simulink model "two_legged_raibert_hopper"  (R2014a)
settings: Solver=FixedStepDiscrete  StartTime=0.0  StopTime=inf  FixedStep=sample_time  RelTol=1e-3
undefined symbols (not defined in the file): A1_notch_f1, A2_notch_f1, A_lpf_accel, A_lpf_dtau, B1_lpf_accel, B1_lpf_dtau, B1_notch_f1, B2_lpf_accel, B2_lpf_dtau, B2_notch_f1, boom_height, boom_mount_angle, boom_mount_to_center_diagonal, boom_mount_to_com, contact_threshold, control_start_time, desired_torso_angle, DiscIntNeverNeededParam, dt_thrust, dx_avg_desired, dx_avg_samples, dx_desired_step, extra_leg_damping, F_thrust, fcut_contact, g, i_limit_lateral, initial_dt, j_segments, k_ff, K_notch_f1, k_placement, k_sea, kd_flight, kd_lateral, kd_leg_angle, kd_leg_length_secondary, kd_sea_torque_flight, kd_sea_torque_stance, kd_torso, kd_virtual, ki_lateral, kp_flight_max, kp_flight_min, kp_lateral, kp_leg_angle, kp_leg_length_secondary, kp_sea_torque_flight, kp_sea_torque_stance, kp_torso, kp_virtual, l0_virtual, l_boom, l_max, l_min, l_retract, l_seg, lambda1, lambda2, lateral_offset ... (+20)
libraries: simulink x14
(part 2 of 2)

== system two_legged_raibert_hopper/Control/Behavior Control/Lateral PID Control/spherical_correction_angle ==
  q_cmu : Inport
  Selector : Selector  InputPortWidth=13  Indices=[11]
  Sum1 : Sum  Inputs=|+-
  Terminator2 : Terminator
  boom_mount_angle : Constant  Value=boom_mount_angle
  lateral_correction : Gain  Gain=180/pi
  lateral_correction [rad] : Outport
  wires:
  Sum1/1 -> lateral_correction/1, lateral_correction [rad]/1
  Selector/1 -> Sum1/1  "qBoomRoll"
  q_cmu/1 -> Selector/1
  boom_mount_angle/1 -> Sum1/2
  lateral_correction/1 -> Terminator2/1

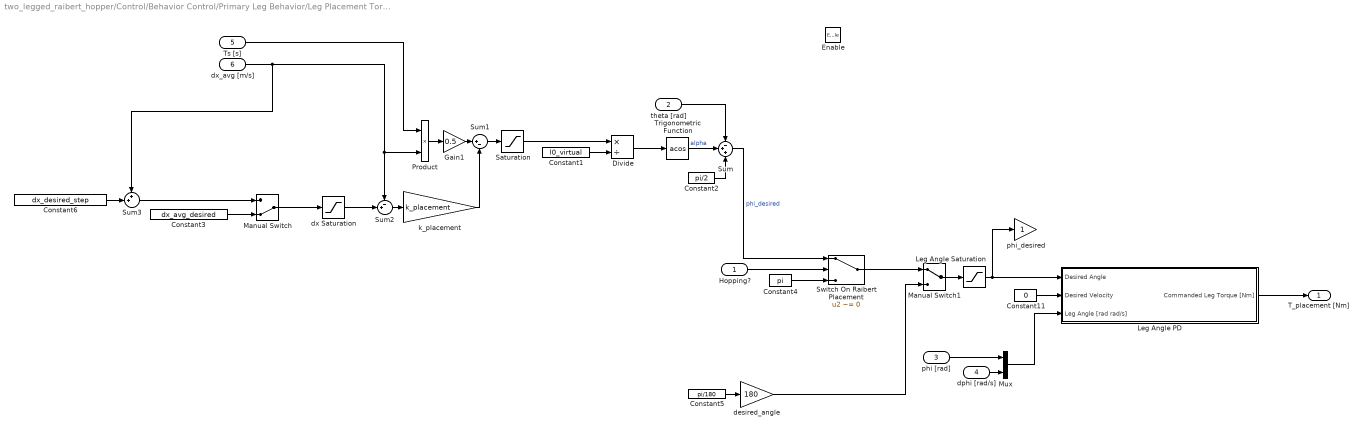
== system two_legged_raibert_hopper/Control/Behavior Control/Primary Leg Behavior/Leg Placement Torque ==
  Hopping? : Inport
  theta [rad] : Inport  Port=2
  phi [rad] : Inport  Port=3
  dphi [rad/s] : Inport  Port=4
  Ts [s] : Inport  Port=5
  dx_avg [m/s] : Inport  Port=6
  Enable : EnablePort  StatesWhenEnabling=reset
  Constant1 : Constant  Value=l0_virtual
  Constant11 : Constant  Value=0
  Constant2 : Constant  Value=pi/2
  Constant3 : Constant  Value=dx_avg_desired
  Constant4 : Constant  Value=pi
  Constant5 : Constant  Value=pi/180
  Constant6 : Constant  Value=dx_desired_step
  Divide : Product  Inputs=*/
  Gain1 : Gain  Gain=0.5
  Leg Angle PD : Subsystem
  Leg Angle Saturation : Saturate  UpperLimit=max_leg_angle  LowerLimit=min_leg_angle
      settings: AttributesFormatString=Hi: %<UpperLimit>\nLo: %<LowerLimit>
  Manual Switch : ManualSwitch  CurrentSetting=0
  Manual Switch1 : ManualSwitch
  Mux : Mux  Inputs=2
  Product : Product
  Saturation : Saturate  UpperLimit=x_limit  LowerLimit=-x_limit
      settings: AttributesFormatString=Hi: %<UpperLimit>\nLo: %<LowerLimit>
  Sum : Sum  Inputs=-++
  Sum1 : Sum  Inputs=|+-
  Sum2 : Sum  Inputs=-+|
  Sum3 : Sum  Inputs=++|
  Switch On Raibert Placement : Switch  Criteria=u2 ~= 0
  Trigonometric Function : Trigonometry  Operator=acos
  desired_angle : Gain  Gain=180
  dx Saturation : Saturate  UpperLimit=dx_avg_desired  LowerLimit=0
      settings: AttributesFormatString=Hi: %<UpperLimit>\nLo: %<LowerLimit>
  k_placement : Gain  Gain=k_placement
  phi_desired : Gain
  T_placement [Nm] : Outport  OutputWhenDisabled=reset  InitialOutput=[0]
  wires:
  Constant11/1 -> Leg Angle PD/2(Desired Velocity)
  Mux/1 -> Leg Angle PD/3(Leg Angle [rad rad/s])
  Leg Angle PD/1(Commanded Leg Torque [Nm]) -> T_placement [Nm]/1
  phi [rad]/1 -> Mux/1
  dphi [rad/s]/1 -> Mux/2
  Ts [s]/1 -> Product/1
  Product/1 -> Gain1/1
  Gain1/1 -> Sum1/1
  Saturation/1 -> Divide/1
  Constant1/1 -> Divide/2
  Trigonometric Function/1 -> Sum/2  "alpha"
  Constant2/1 -> Sum/3
  theta [rad]/1 -> Sum/1
  Sum/1 -> Switch On Raibert Placement/1  "phi_desired"
  Sum1/1 -> Saturation/1
  k_placement/1 -> Sum1/2
  Sum2/1 -> k_placement/1
  dx Saturation/1 -> Sum2/2
  Constant4/1 -> Switch On Raibert Placement/3
  Hopping?/1 -> Switch On Raibert Placement/2
  Leg Angle Saturation/1 -> phi_desired/1, Leg Angle PD/1(Desired Angle)
  Constant5/1 -> desired_angle/1
  Manual Switch/1 -> dx Saturation/1
  Constant3/1 -> Manual Switch/2
  dx_avg [m/s]/1 -> Sum3/1, Sum2/1, Product/2
  Constant6/1 -> Sum3/2
  Sum3/1 -> Manual Switch/1
  Divide/1 -> Trigonometric Function/1
  Switch On Raibert Placement/1 -> Manual Switch1/1
  desired_angle/1 -> Manual Switch1/2
  Manual Switch1/1 -> Leg Angle Saturation/1

== system two_legged_raibert_hopper/Control/Behavior Control/Primary Leg Behavior/Leg Thrust ==
  Enable : EnablePort  StatesWhenEnabling=reset  ShowOutputPort=on
  F_thrust : Gain  Gain=F_thrust
  Thrust Timer : Subsystem
  thrust period? : simulink/Logic and Bit Operations/Compare To Constant  relop=<=  const=dt_thrust  OutDataTypeStr=uint8
  Thrust [N] : Outport  OutputWhenDisabled=reset  InitialOutput=[0]
  wires:
  F_thrust/1 -> Thrust [N]/1
  Thrust Timer/1(timer [s]) -> thrust period?/1
  Enable/1 -> Thrust Timer/Enable
  thrust period?/1 -> F_thrust/1

== system two_legged_raibert_hopper/Control/Behavior Control/Primary Leg Behavior/Trunk Balance PD Compensation ==
  Torso Pitch [rad rad/s] : Inport
  Enable : EnablePort  StatesWhenEnabling=reset
  Constant2 : Constant  Value=0
  Demux : Demux  Outputs=2
  Derivative Gain : Gain  Gain=kd_torso
  Gain1 : Gain  Gain=-1
  Proportional Gain : Gain  Gain=kp_torso
  Reference Lean [rad] : Constant  Value=desired_torso_angle
  Sum1 : Sum  Inputs=|+-
  Sum4 : Sum  Inputs=|+-
  Sum5 : Sum
  Commanded Torque [Nm] : Outport  OutputWhenDisabled=reset  InitialOutput=[0]
  wires:
  Gain1/1 -> Commanded Torque [Nm]/1
  Sum1/1 -> Derivative Gain/1
  Proportional Gain/1 -> Sum5/1
  Derivative Gain/1 -> Sum5/2
  Torso Pitch [rad rad/s]/1 -> Demux/1
  Sum4/1 -> Proportional Gain/1
  Demux/1 -> Sum4/2
  Reference Lean [rad]/1 -> Sum4/1
  Constant2/1 -> Sum1/1
  Demux/2 -> Sum1/2
  Sum5/1 -> Gain1/1

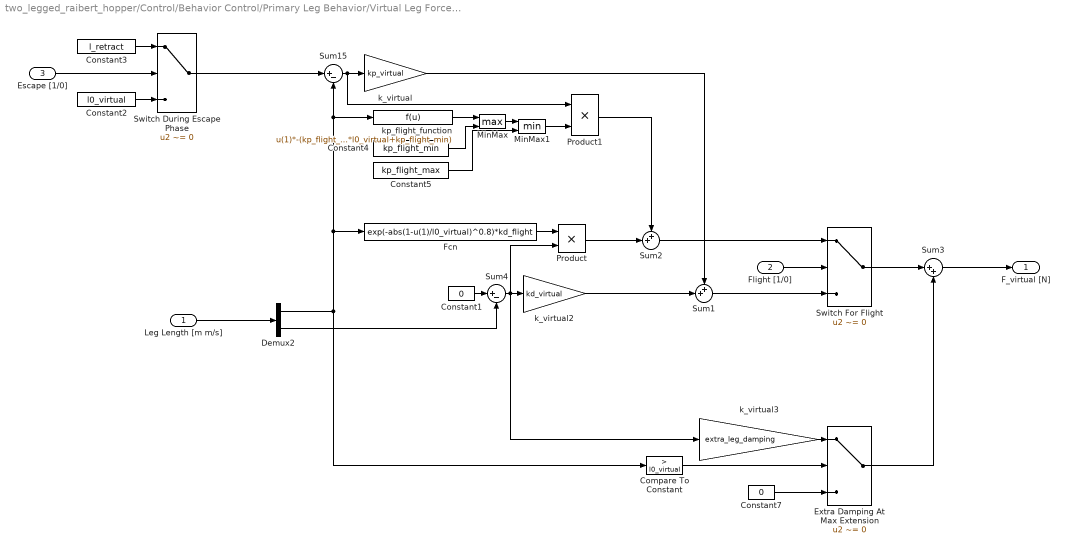
== system two_legged_raibert_hopper/Control/Behavior Control/Primary Leg Behavior/Virtual Leg Force and Swing Leg Retraction ==
  Leg Length [m m/s] : Inport
  Flight [1/0] : Inport  Port=2
  Escape [1/0] : Inport  Port=3
  Compare To Constant : simulink/Logic and Bit Operations/Compare To Constant  relop=>  const=l0_virtual  OutDataTypeStr=boolean
  Constant1 : Constant  Value=0
  Constant2 : Constant  Value=l0_virtual
  Constant3 : Constant  Value=l_retract
  Constant4 : Constant  Value=kp_flight_min
  Constant5 : Constant  Value=kp_flight_max
  Constant7 : Constant  Value=0
  Demux2 : Demux  Outputs=2
  Extra Damping At Max Extension : Switch  Criteria=u2 ~= 0
  Fcn : Fcn  Expr=exp(-abs(1-u(1)/l0_virtual)^0.8)*kd_flight
  MinMax : MinMax  Function=max  Inputs=2
  MinMax1 : MinMax  Inputs=2
  Product : Product
  Product1 : Product
  Sum1 : Sum  Inputs=++|
  Sum15 : Sum  Inputs=|+-
  Sum2 : Sum  Inputs=++|
  Sum3 : Sum  Inputs=|++
  Sum4 : Sum  Inputs=|+-
  Switch During Escape Phase : Switch  Criteria=u2 ~= 0
  Switch For Flight : Switch  Criteria=u2 ~= 0
  k_virtual : Gain  Gain=kp_virtual
  k_virtual2 : Gain  Gain=kd_virtual
  k_virtual3 : Gain  Gain=extra_leg_damping
  kp_flight_function : Fcn  Expr=u(1)*-(kp_flight_max - kp_flight_min)/(l0_virtual - l_min)+((kp_flight_max - kp_flight_min)/(l0_virtual - l_min)*l0_virtual+kp_flight_min)
  F_virtual [N] : Outport
  wires:
  Sum2/1 -> Switch For Flight/1
  Switch For Flight/1 -> Sum3/1
  Product/1 -> Sum2/2
  Constant3/1 -> Switch During Escape Phase/1
  Constant2/1 -> Switch During Escape Phase/3
  Escape [1/0]/1 -> Switch During Escape Phase/2
  Flight [1/0]/1 -> Switch For Flight/2
  k_virtual2/1 -> Sum1/2
  Sum4/1 -> k_virtual3/1, Product/2, k_virtual2/1
  k_virtual/1 -> Sum1/1
  Demux2/2 -> Sum4/2
  Constant1/1 -> Sum4/1
  Sum1/1 -> Switch For Flight/3
  Demux2/1 -> kp_flight_function/1, Sum15/2, Fcn/1, Compare To Constant/1
  Leg Length [m m/s]/1 -> Demux2/1
  Sum15/1 -> Product1/1, k_virtual/1
  Fcn/1 -> Product/1
  kp_flight_function/1 -> MinMax/1
  Product1/1 -> Sum2/1
  MinMax/1 -> MinMax1/1
  Constant4/1 -> MinMax/2
  MinMax1/1 -> Product1/2
  Constant5/1 -> MinMax1/2
  Switch During Escape Phase/1 -> Sum15/1
  Compare To Constant/1 -> Extra Damping At Max Extension/2
  Constant7/1 -> Extra Damping At Max Extension/3
  Extra Damping At Max Extension/1 -> Sum3/2
  Sum3/1 -> F_virtual [N]/1
  k_virtual3/1 -> Extra Damping At Max Extension/1

== system two_legged_raibert_hopper/Control/Behavior Control/Primary Secondary Leg Swap/Toggle ==
  Trigger : TriggerPort  TriggerType=falling  PortDimensions=1
  Logical Operator : Logic  Operator=NOT  AllPortsSameDT=off  OutDataTypeStr=boolean
  Memory : Memory  X0=1  InheritSampleTime=on
  "[1/0]" : Outport  InitialOutput=[1]
  wires:
  Memory/1 -> Logical Operator/1
  Logical Operator/1 -> Memory/1, "[1/0]"/1

== system two_legged_raibert_hopper/Control/Behavior Control/Secondary Leg Behavior/Leg Angle PD ==
  Desired Angle : Inport
  Desired Velocity : Inport  Port=2
  Leg Angle [rad rad/s] : Inport  Port=3
  Demux1 : Demux  Outputs=2
  Gain6 : Gain  Gain=kp_leg_angle
  Gain7 : Gain  Gain=kd_leg_angle
  Sum7 : Sum  Inputs=|+-
  Sum8 : Sum  Inputs=|+-
  Sum9 : Sum  Inputs=|++
  Commanded Leg Torque [Nm] : Outport
  wires:
  Leg Angle [rad rad/s]/1 -> Demux1/1
  Demux1/2 -> Sum8/2
  Gain7/1 -> Sum9/2
  Desired Angle/1 -> Sum7/1
  Sum8/1 -> Gain7/1
  Desired Velocity/1 -> Sum8/1
  Sum9/1 -> Commanded Leg Torque [Nm]/1
  Demux1/1 -> Sum7/2
  Sum7/1 -> Gain6/1
  Gain6/1 -> Sum9/1

== system two_legged_raibert_hopper/Control/Behavior Control/Secondary Leg Behavior/Leg Length PD ==
  Desired Length : Inport
  Desired Velocity : Inport  Port=2
  Leg Length [m m/s] : Inport  Port=3
  Demux1 : Demux  Outputs=2
  Sum7 : Sum  Inputs=|+-
  Sum8 : Sum  Inputs=|+-
  Sum9 : Sum
  kd_leg_length_secondary : Gain  Gain=kd_leg_length_secondary
  kp_leg_length_secondary : Gain  Gain=kp_leg_length_secondary
  Commanded Force [N] : Outport
  wires:
  kp_leg_length_secondary/1 -> Sum9/1
  Sum7/1 -> kp_leg_length_secondary/1
  Demux1/1 -> Sum7/2  "l_measured"
  Sum9/1 -> Commanded Force [N]/1
  Desired Velocity/1 -> Sum8/1
  Sum8/1 -> kd_leg_length_secondary/1
  Desired Length/1 -> Sum7/1
  kd_leg_length_secondary/1 -> Sum9/2
  Demux1/2 -> Sum8/2  "l_dot_measured"
  Leg Length [m m/s]/1 -> Demux1/1

== system two_legged_raibert_hopper/Control/Behavior Control/Velocity Estimation/Recursive Moving Average ==
  dx [m/s] : Inport
  Delay : Delay  DelayLength=dx_avg_samples  InitialCondition=0  UseCircularBuffer=on  SampleTime=sample_time
  Gain : Gain  Gain=1/dx_avg_samples
  Sum : Sum  Inputs=-++
  Unit Delay : UnitDelay  SampleTime=sample_time
  dx_avg [m/s] : Outport
  wires:
  dx [m/s]/1 -> Delay/1, Sum/2
  Sum/1 -> Gain/1, Unit Delay/1
  Delay/1 -> Sum/1
  Gain/1 -> dx_avg [m/s]/1
  Unit Delay/1 -> Sum/3

== system two_legged_raibert_hopper/Control/Behavior Control/Primary Leg Behavior/Leg Placement Torque/Leg Angle PD ==
  Desired Angle : Inport
  Desired Velocity : Inport  Port=2
  Leg Angle [rad rad/s] : Inport  Port=3
  Demux1 : Demux  Outputs=2
  Sum7 : Sum  Inputs=|+-
  Sum8 : Sum  Inputs=|+-
  Sum9 : Sum
  kd_leg_angle : Gain  Gain=kd_leg_angle
  kp_leg_angle : Gain  Gain=kp_leg_angle
  Commanded Leg Torque [Nm] : Outport
  wires:
  Leg Angle [rad rad/s]/1 -> Demux1/1
  Demux1/2 -> Sum8/2
  kd_leg_angle/1 -> Sum9/2
  Desired Angle/1 -> Sum7/1
  Sum8/1 -> kd_leg_angle/1
  Desired Velocity/1 -> Sum8/1
  Sum9/1 -> Commanded Leg Torque [Nm]/1
  Demux1/1 -> Sum7/2
  Sum7/1 -> kp_leg_angle/1
  kp_leg_angle/1 -> Sum9/1

== system two_legged_raibert_hopper/Control/Behavior Control/Primary Leg Behavior/Leg Thrust/Thrust Timer ==
  Enable : EnablePort  StatesWhenEnabling=reset  ShowOutputPort=on
  Constant : Constant
  Discrete-Time Integrator : DiscreteIntegrator  IntegratorMethod=Accumulation: Forward Euler  gainval=sample_time  ExternalReset=rising  SampleTime=sample_time  ICPrevOutput=DiscIntNeverNeededParam  ICPrevScaledInput=DiscIntNeverNeededParam
  timer [s] : Outport  InitialOutput=[0]
  wires:
  Discrete-Time Integrator/1 -> timer [s]/1
  Enable/1 -> Discrete-Time Integrator/2
  Constant/1 -> Discrete-Time Integrator/1

== stateflow chart two_legged_raibert_hopper/Control/Behavior Control/Primary Leg Behavior/Raibert  Hopper State Machine ==
  state Loading
    entry: placement = 0;
    entry: posture = 0;
    entry: thrust = 0;
    entry: flight = 0;
    entry: escape = 0;
  state Compression
    entry: placement = 0;
    entry: posture = 1;
    entry: thrust = 0;
    entry: flight = 0;
    entry: escape = 0;
  state Thrust
    entry: placement = 0;
    entry: posture = 1;
    entry: thrust = 1;
    entry: flight = 0;
    entry: escape = 0;
  state Unloading
    entry: placement = 0;
    entry: posture = 0;
    entry: thrust = 1;
    entry: flight = 0;
    entry: escape = 0;
  state Escape
    entry: placement = 0;
    entry: posture = 0;
    entry: thrust = 0;
    entry: flight = 1;
    entry: escape = 1;
  state Flight
    entry: placement = 1;
    entry: posture = 0;
    entry: thrust = 0;
    entry: flight = 1;
    entry: escape = 0;
  (junction 91) -> Loading
  Loading -> (junction 130) [order 2] : [Fy < contact_threshold]
  (junction 93) -> (junction 91)
  (junction 130) -> (junction 128)
  Loading -> Compression [order 1] : [Fy > loaded_threshold]
  (junction 115) -> Compression
  (junction 118) -> (junction 115)
  Compression -> Thrust : [dl >= 0 && dl_prev < 0]
  Thrust -> Unloading [order 1] : [Fy < loaded_threshold]
  Thrust -> (junction 102) [order 2] : [l > l_max]
  (junction 102) -> (junction 100)
  (junction 122) -> (junction 118)
  Unloading -> Escape [order 1] : [Fy < contact_threshold || l > l_max]
  Unloading -> (junction 122) [order 2] : [Fy > loaded_threshold]
  Escape -> Flight : after(t_flight,sec)
  (junction 100) -> Escape
  (default) -> Flight
  Flight -> (junction 93) : [Fy > contact_threshold]
  (junction 128) -> Flight
  data: flight output; escape output; thrust output; posture output; l input; dl input; dl_prev input; Fy input; t_flight parameter; placement output; l_max parameter; contact_threshold parameter; loaded_threshold parameter

== matlab function two_legged_raibert_hopper/Control/Behavior Control/Torque Distribution Right/Motor Torque Saturation Optimization ==
  data: x1s input; t1 output; x2s input; lambda1 parameter; lambda2 parameter; LEG_MTR_MAX_TORQUE parameter; t2 output
% Optimal leg motor torque distribution
function [t1, t2] = distribute_torque(x1s, x2s, lambda1, lambda2, LEG_MTR_MAX_TORQUE)

s = LEG_MTR_MAX_TORQUE;

% possible solutions
x1 = [                                                      x1s;
                                                            0;
                                                            s;
                                                            0;
                                                           -s;
  (lambda2*s + lambda1*x1s - lambda2*x2s)/(lambda1 + lambda2);
  (lambda1*x1s - lambda2*s + lambda2*x2s)/(lambda1 + lambda2);
  (lambda2*s + lambda1*x1s + lambda2*x2s)/(lambda1 + lambda2);
 -(lambda2*s - lambda1*x1s + lambda2*x2s)/(lambda1 + lambda2)];
 
x2 = [                                                      x2s;
                                                            s;
                                                            0;
                                                           -s;
                                                            0;
  (lambda1*s - lambda1*x1s + lambda2*x2s)/(lambda1 + lambda2);
  (lambda1*s + lambda1*x1s + lambda2*x2s)/(lambda1 + lambda2);
  (lambda1*x1s - lambda1*s + lambda2*x2s)/(lambda1 + lambda2);
 -(lambda1*s + lambda1*x1s - lambda2*x2s)/(lambda1 + lambda2)];

% test constraints
c1 = s - x1 - x2 >= 0;
c2 = s + x1 + x2 >= 0;
c3 = s - x1 + x2 >= 0;
c4 = s + x1 - x2 >= 0;
constraints = c1 & c2 & c3 & c4;

% objective function to maximize
f = -lambda1*(x1-x1s).^2-lambda2*(x2-x2s).^2;
satisfied = find(constraints);
[~,I] = max(f(satisfied));

t1 = x1(satisfied(I));
t2 = x2(satisfied(I));

== matlab function two_legged_raibert_hopper/Control/Behavior Control/Velocity Estimation/dx_from_yaw_and_roll ==
  data: qRoll input; dx output; dqYaw input; dqPitch input; l_boom parameter; boom_mount_to_center_diagonal parameter; boom_mount_to_com parameter
function dx = fcn(qRoll, dqYaw, dqPitch, l_boom, boom_mount_to_center_diagonal, boom_mount_to_com)
    dx = (l_boom+boom_mount_to_center_diagonal)*(dqYaw*cos(qRoll)) - dqPitch*boom_mount_to_com;

== matlab function two_legged_raibert_hopper/Control/Behavior Control/Torque Distribution Left/Motor Torque Saturation Optimization ==
  data: x1s input; t1 output; x2s input; lambda1 parameter; lambda2 parameter; LEG_MTR_MAX_TORQUE parameter; t2 output
% Optimal leg motor torque distribution
function [t1, t2] = distribute_torque(x1s, x2s, lambda1, lambda2, LEG_MTR_MAX_TORQUE)

s = LEG_MTR_MAX_TORQUE;

% possible solutions
x1 = [                                                      x1s;
                                                            0;
                                                            s;
                                                            0;
                                                           -s;
  (lambda2*s + lambda1*x1s - lambda2*x2s)/(lambda1 + lambda2);
  (lambda1*x1s - lambda2*s + lambda2*x2s)/(lambda1 + lambda2);
  (lambda2*s + lambda1*x1s + lambda2*x2s)/(lambda1 + lambda2);
 -(lambda2*s - lambda1*x1s + lambda2*x2s)/(lambda1 + lambda2)];
 
x2 = [                                                      x2s;
                                                            s;
                                                            0;
                                                           -s;
                                                            0;
  (lambda1*s - lambda1*x1s + lambda2*x2s)/(lambda1 + lambda2);
  (lambda1*s + lambda1*x1s + lambda2*x2s)/(lambda1 + lambda2);
  (lambda1*x1s - lambda1*s + lambda2*x2s)/(lambda1 + lambda2);
 -(lambda1*s + lambda1*x1s - lambda2*x2s)/(lambda1 + lambda2)];

% test constraints
c1 = s - x1 - x2 >= 0;
c2 = s + x1 + x2 >= 0;
c3 = s - x1 + x2 >= 0;
c4 = s + x1 - x2 >= 0;
constraints = c1 & c2 & c3 & c4;

% objective function to maximize
f = -lambda1*(x1-x1s).^2-lambda2*(x2-x2s).^2;
satisfied = find(constraints);
[~,I] = max(f(satisfied));

t1 = x1(satisfied(I));
t2 = x2(satisfied(I));
